simulink model "Sudarshan_2_lab_6"  (R2022b)
settings: Solver=VariableStepAuto  StartTime=0.0  StopTime=10  RelTol=1e-3
settings Model: Creator=year2  LastModifiedBy=year2

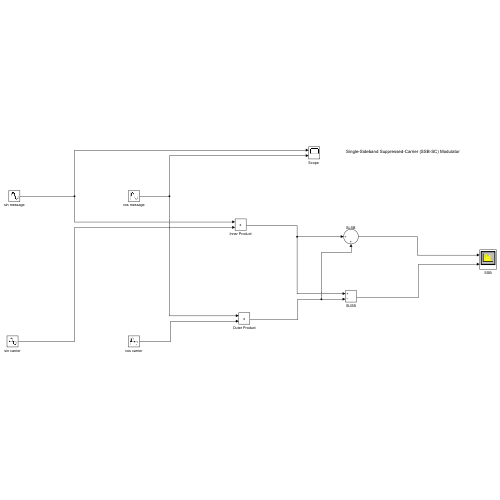
[thumbnail: Simulink's stored preview of the top-level diagram]
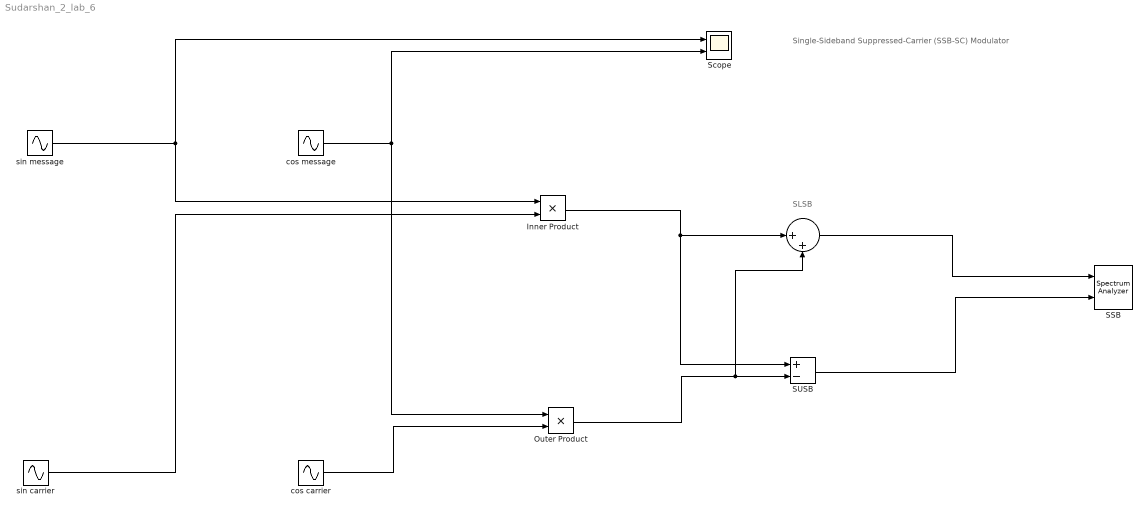
== system Sudarshan_2_lab_6 ==
  note: Single-Sideband Suppressed-Carrier (SSB-SC) Modulator
  note: SLSB
  " " : Sum  Inputs=|++
  Inner Product : Product
  Outer Product : Product
  SSB : SpectrumAnalyzer  NumInputPorts=2
  SUSB : Sum  Inputs=+-
  "Scope " : Scope  NumInputPorts=2
  cos carrier : Sin  Frequency=2*pi*10000  Phase=pi/2  SampleTime=1e-5
  cos message : Sin  Frequency=2*pi*1000  Phase=pi/2  SampleTime=1e-5
  sin carrier : Sin  Frequency=2*pi*10000  SampleTime=1e-5
  sin message : Sin  Frequency=2*pi*1000  SampleTime=1e-5
  wires:
  sin message/1 -> Inner Product/1, "Scope "/1
  cos message/1 -> "Scope "/2, Outer Product/1
  sin carrier/1 -> Inner Product/2
  cos carrier/1 -> Outer Product/2
  Inner Product/1 -> SUSB/1, " "/1
  Outer Product/1 -> SUSB/2, " "/2
  " "/1 -> SSB/1
  SUSB/1 -> SSB/2
